simulink model "robot3_CTC_sin"  (R2023b)
settings: Solver=FixedStepAuto  StartTime=0.0  StopTime=10.0  RelTol=1e-3
undefined symbols (not defined in the file): Coriolis3, Dhat3, Dinv3, Gravity3
libraries: simulink x1
settings Model: Creator=사용자  LastModifiedBy=사용자

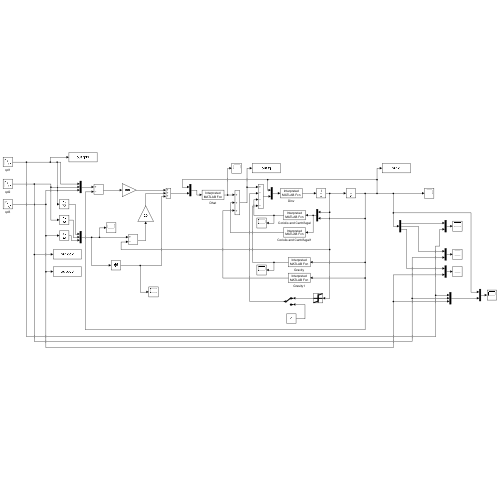
[thumbnail: Simulink's stored preview of the top-level diagram]
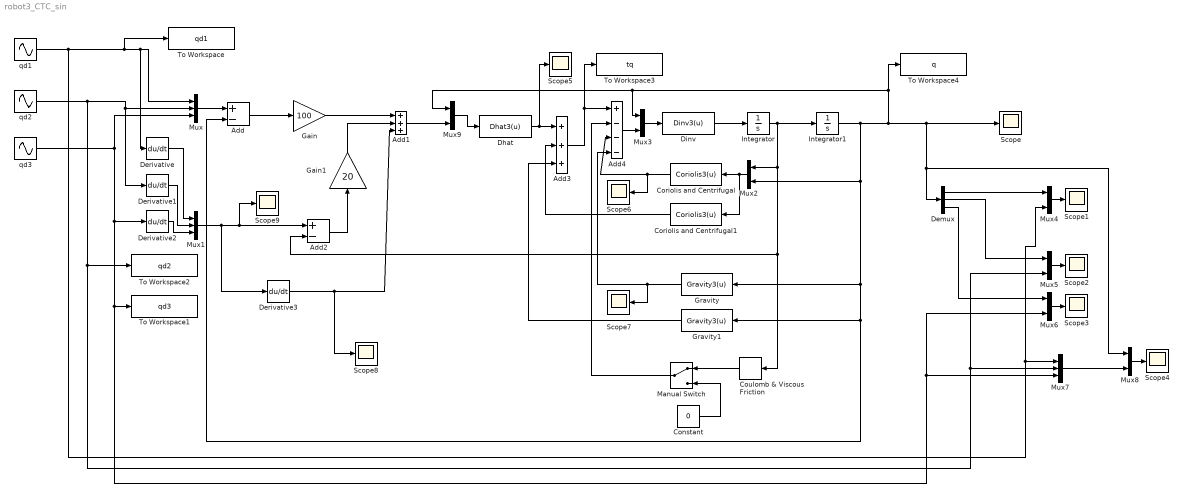
== system robot3_CTC_sin ==
  Add : Sum  Inputs=+-
  Add1 : Sum  Inputs=+++
  Add2 : Sum  Inputs=+-
  Add3 : Sum  Inputs=+++
  Add4 : Sum  Inputs=+---
  Constant : Constant  Value=0
  Coriolis and Centrifugal : MATLABFcn  MATLABFcn=Coriolis3(u)  OutputDimensions=3  Output1D=off
  Coriolis and Centrifugal1 : MATLABFcn  MATLABFcn=Coriolis3(u)  OutputDimensions=3  Output1D=off
  Coulomb & Viscous Friction : simulink/Discontinuities/Coulomb & Viscous Friction  offset=5  gain=3
  Demux : Demux  Outputs=3
  Derivative{,1..3} (4 alike) : Derivative
  Dhat : MATLABFcn  MATLABFcn=Dhat3(u)  OutputDimensions=3  Output1D=off
  Dinv : MATLABFcn  MATLABFcn=Dinv3(u)  OutputDimensions=3  Output1D=off
  Gain : Gain  Gain=100
  Gain1 : Gain  Gain=20
  Gravity : MATLABFcn  MATLABFcn=Gravity3(u)  OutputDimensions=3  Output1D=off
  Gravity1 : MATLABFcn  MATLABFcn=Gravity3(u)  OutputDimensions=3  Output1D=off
  Integrator : Integrator  InitialCondition=[0;0;0];
  Integrator1 : Integrator  InitialCondition=[pi/2;pi/2;-pi/2]
  Manual Switch : ManualSwitch
  Mux : Mux  Inputs=3
  Mux1 : Mux  Inputs=3
  Mux{2..6,8..9} (7 alike) : Mux  Inputs=2
  Mux7 : Mux  Inputs=3
  Scope{,1..9} (10 alike) : Scope
  To Workspace : ToWorkspace  VariableName=qd1  SaveFormat=Timeseries  SampleTime=0.001
  To Workspace1 : ToWorkspace  VariableName=qd3  SaveFormat=Timeseries  SampleTime=0.001
  To Workspace2 : ToWorkspace  VariableName=qd2  SaveFormat=Timeseries  SampleTime=0.001
  To Workspace3 : ToWorkspace  VariableName=tq  SaveFormat=Timeseries  SampleTime=0.001
  To Workspace4 : ToWorkspace  VariableName=q  SaveFormat=Timeseries  SampleTime=0.001
  qd1 : Sin  Bias=pi/2  SampleTime=0
  qd2 : Sin  Amplitude=-1  Bias=pi/2  SampleTime=0
  qd3 : Sin  Bias=-pi/2  SampleTime=0
  wires:
  Mux/1 -> Add/1
  qd3/1 -> Mux/3, Mux6/2, Mux7/3, To Workspace1/1, Derivative2/1
  Derivative/1 -> Mux1/1
  Derivative1/1 -> Mux1/2
  Derivative2/1 -> Mux1/3
  Mux1/1 -> Derivative3/1, Scope9/1, Add2/1
  Add2/1 -> Gain1/1
  Gain/1 -> Add1/1
  Gain1/1 -> Add1/2
  Add/1 -> Gain/1
  Dinv/1 -> Integrator/1
  Mux2/1 -> Coriolis and Centrifugal/1, Coriolis and Centrifugal1/1
  Integrator/1 -> Coulomb & Viscous Friction/1, Add2/2, Mux2/1, Integrator1/1
  Integrator1/1 -> Mux2/2, Gravity/1, Gravity1/1, Add/2, Demux/1, Mux8/1, Scope/1, Mux3/1, Mux9/1, To Workspace4/1
  Mux4/1 -> Scope1/1
  Mux5/1 -> Scope2/1
  Mux6/1 -> Scope3/1
  Demux/1 -> Mux4/1
  Demux/2 -> Mux5/1
  Demux/3 -> Mux6/1
  qd1/1 -> Mux4/2, Mux7/1, To Workspace/1, Derivative/1, Mux/1
  qd2/1 -> Mux5/2, Mux7/2, To Workspace2/1, Derivative1/1, Mux/2
  Mux7/1 -> Mux8/2
  Mux8/1 -> Scope4/1
  Derivative3/1 -> Scope8/1, Add1/3
  Add1/1 -> Mux9/2
  Mux9/1 -> Dhat/1
  Mux3/1 -> Dinv/1
  Add4/1 -> Mux3/2
  Dhat/1 -> Scope5/1, Add3/1
  Coriolis and Centrifugal1/1 -> Add3/2
  Gravity1/1 -> Add3/3
  Coriolis and Centrifugal/1 -> Scope6/1, Add4/3
  Gravity/1 -> Scope7/1, Add4/4
  Add3/1 -> To Workspace3/1, Add4/1
  Constant/1 -> Manual Switch/2
  Manual Switch/1 -> Add4/2
  Coulomb & Viscous Friction/1 -> Manual Switch/1
